simulink model "validacao_2a_ordem"  (R2021a)
settings: Solver=ode4  StartTime=0.0  StopTime=t(end)  FixedStep=1e-3  RelTol=1e-3
values from neighbouring files (symbols this model uses):
  A = [ -Ra/La -kg/(kt*La); (ka*kt)/j -f/j]    [parametros_2a_ordem.m]
  B = [1/La ; 0]    [parametros_2a_ordem.m]
  C1 = [1 0]    [parametros_2a_ordem.m]
  C2 = [0 1]    [parametros_2a_ordem.m]
  D = 0    [parametros_2a_ordem.m]
  Ia = Ia - Ia(1)    [parametros_2a_ordem.m]
  Vt = Vt - Vt(1)    [parametros_2a_ordem.m]
settings Model: Creator=Gabriel  LastModifiedBy=Lucas Bussoli
settings SolverCC: AlgebraicLoopSolver=TrustRegion
settings DebuggingCC: SFMachineParentedDataDiag=warning
settings SFSimCC: CustomCodeUndefinedFunction=UseInterfaceOnly

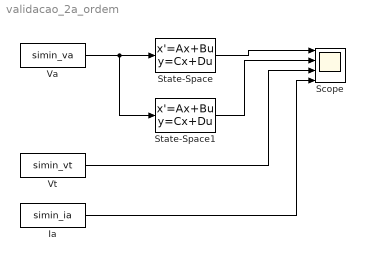
== system validacao_2a_ordem ==
  Ia : FromWorkspace  VariableName=simin_ia
  Scope : Scope  NumInputPorts=4
  State-Space : StateSpace  A=A  B=B  C=C1  D=D  InitialCondition=[Ia(1), Vt(1)]
  State-Space1 : StateSpace  A=A  B=B  C=C2  D=D  InitialCondition=[Ia(1), Vt(1)]
  Va : FromWorkspace  VariableName=simin_va
  Vt : FromWorkspace  VariableName=simin_vt
  wires:
  State-Space/1 -> Scope/1
  Va/1 -> State-Space1/1, State-Space/1
  State-Space1/1 -> Scope/2
  Vt/1 -> Scope/3
  Ia/1 -> Scope/4
